simulink model "Winkelsensor"  (R2022a)
settings: Solver=ode3  StartTime=0.0  StopTime=10.0  FixedStep=0.01  RelTol=1e-3  EnableMultiTasking=on
settings Model: Creator=60251  LastModifiedBy=yufu

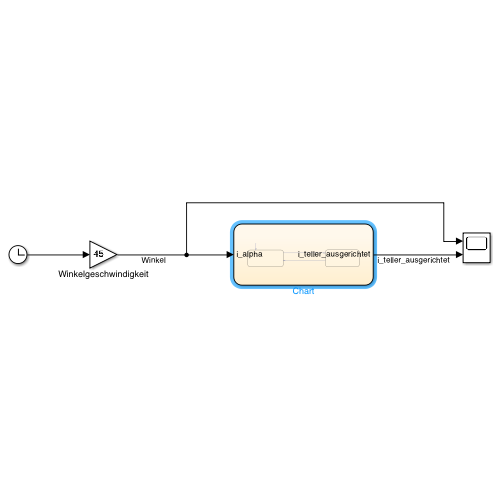
[thumbnail: Simulink's stored preview of the top-level diagram]
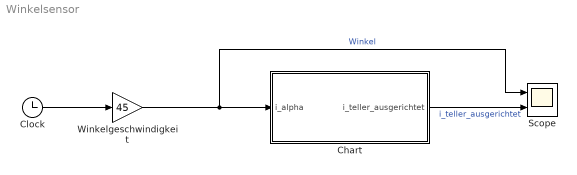
== system Winkelsensor ==
  Chart : Stateflow chart  TreatAsAtomicUnit=on
  Clock : Clock
  Scope : Scope  NumInputPorts=2
  Winkelgeschwindigkeit : Gain  Gain=45
  wires:
  Clock/1 -> Winkelgeschwindigkeit/1
  Winkelgeschwindigkeit/1 -> Scope/1, Chart/1(i_alpha)  "Winkel"
  Chart/1(i_teller_ausgerichtet) -> Scope/2  "i_teller_ausgerichtet"

== stateflow chart Winkelsensor/Chart ==
  state eingerichtet
    en: i_teller_ausgerichtet = 0;
  state ausgerichtet
    en: i_teller_ausgerichtet = 1;
    %entry=Eintritt
  (default) -> ausgerichtet
  ausgerichtet -> eingerichtet : [mod(i_alpha+1, 90) > 2]
  eingerichtet -> ausgerichtet : [mod(i_alpha+1, 90) <= 2]
  data: i_alpha input; i_teller_ausgerichtet output
